simulink model "Level2Model"  (R2019a)
settings: Solver=VariableStepAuto  StartTime=0.0  StopTime=10.0  RelTol=1e-3
settings Model: Creator=coeng  LastModifiedBy=coeng

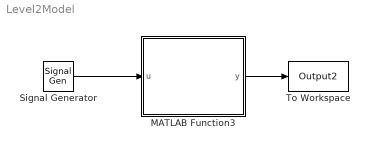
== system Level2Model ==
  MATLAB Function3 : MATLAB Function  TreatAsAtomicUnit=on
  Signal Generator : SignalGenerator  Amplitude=2  Units=rad/sec
  To Workspace : ToWorkspace  VariableName=Output2  SaveFormat=Timeseries  SampleTime=-1
  wires:
  MATLAB Function3/1(y) -> To Workspace/1
  Signal Generator/1 -> MATLAB Function3/1(u)

== matlab function Level2Model/MATLAB Function3 ==
  data: u input; y output; Parameters parameter
function y = T(u, Parameters)
    % T = km*u - Te*dTe;
    km = Parameters.km;
    T = km*u;

y = [T; 0];
